simulink model "backstepping_HW"  (R2023a)
settings: Solver=FixedStepAuto  StartTime=0.0  StopTime=inf  FixedStep=0.001  RelTol=1e-3  EnableMultiTasking=on
values from neighbouring files (symbols this model uses):
  R_p_x = sqrt(2)/2*[-1 1 ... (first row only)    [Init_control.m]
undefined symbols (not defined in the file or in its folder): dev, Main, pwm_output0
libraries: px4Sensorslib x2, simulink x2, px4lib x1
settings Model: SimulationMode=external  ExtModeTrigDuration=10  Creator=ArriGE66  LastModifiedBy=matte
settings SolverCC: PositivePriorityOrder=on
settings OptimizationCC: EnhancedBackFolding=on  PassReuseOutputArgsAs=Individual arguments  ZeroExternalMemoryAtStartup=off  ZeroInternalMemoryAtStartup=off  MaxStackSize=64  OptimizeBlockOrder=speed  DifferentSizesBufferReuse=on  EfficientTunableParamExpr=on
settings DebuggingCC: ParameterTunabilityLossMsg=error
settings HardwareCC: ProdBitPerPointer=32  ProdBitPerSizeT=32  ProdBitPerPtrDiffT=32  ProdLargestAtomicInteger=Long  ProdLargestAtomicFloat=Double  ProdWordSize=32  ProdLongLongMode=on  ProdHWDeviceType=ARM Compatible->ARM Cortex
settings SFSimCC: MATLABDynamicMemAlloc=off  SimTargetLang=C++
settings RTWCC: Description=Embedded Coder  SystemTargetFile=ert.tlc  HardwareBoard=PX4 Cube Orange  TemplateMakefile=ert_default_tmf  Toolchain=GNU Tools for PX4 Autopilots  TargetLang=C++
settings CodeAppCC: ForceParamTrailComments=on  IgnoreCustomStorageClasses=off  OperatorAnnotations=on  SimulinkDataObjDesc=on  SFDataObjDesc=on  InsertBlockDesc=on
settings ERTTargetCC: ExtMode=on  ExtModeTransport=3  ExtModeStaticAlloc=on  ExtModeStaticAllocSize=1024  ExtModeMexFile=ext_xcp  ExtModeMexArgs=1 COM10 3000000  ExtModeIntrfLevel=Level2 - Open

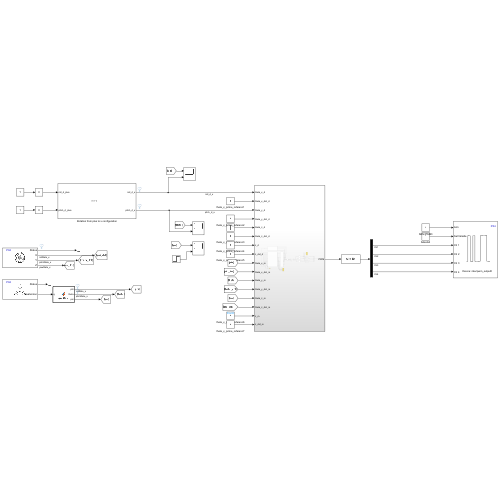
[thumbnail: Simulink's stored preview of the top-level diagram]
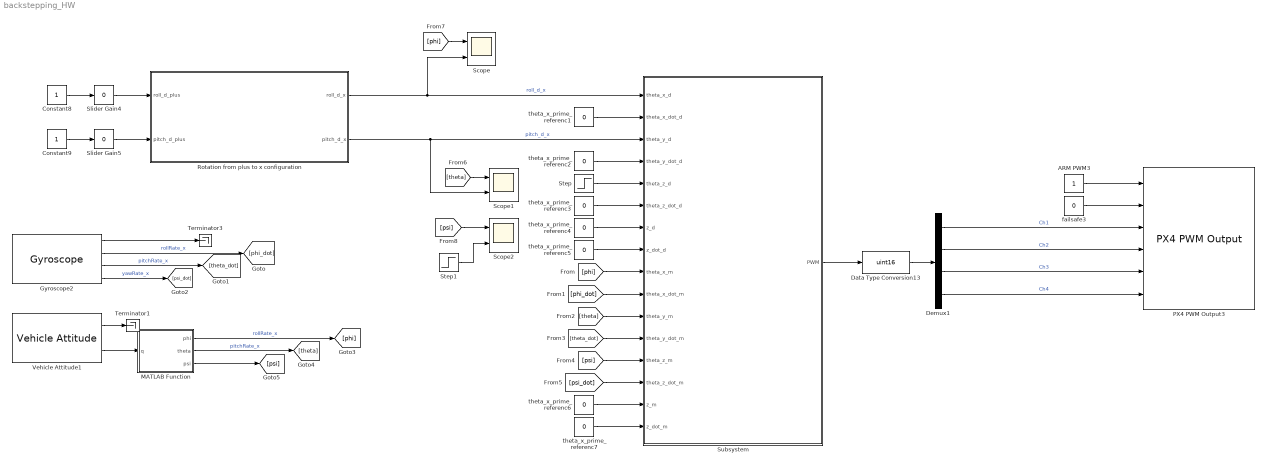
== system backstepping_HW ==
  ARM PWM3 : Constant  OutDataTypeStr=boolean  SampleTime=0.002
  Constant8 : Constant  SampleTime=-1
  Constant9 : Constant  SampleTime=-1
  Data Type Conversion13 : DataTypeConversion  OutDataTypeStr=uint16  SaturateOnIntegerOverflow=off  RndMeth=Floor
  Demux1 : Demux
  Gyroscope2 : px4Sensorslib/Gyroscope  uorbTimeStamp=off  BlockingMode=off  BlockTimeout=1e-3  sampleTime=0.002
  MATLAB Function : MATLAB Function  TreatAsAtomicUnit=on
  PX4 PWM Output3 : px4lib/PX4 PWM Output  pwmDevice=Main (/dev/pwm_output0)  pwmChannel1_=on  pwmChannel2_=on  pwmChannel3_=on  pwmChannel4_=on  pwmChannel5_=off  pwmChannel6_=off  pwmChannel7_=off  pwmChannel8_=off  forceTerminateFailsafe=off  outputErrorStatus=off
  Rotation from plus to x configuration : Subsystem
      mask Display: image('rotation_matrix.jpg');
  Scope : Scope  NumInputPorts=2
  Scope1 : Scope  NumInputPorts=2
  Scope2 : Scope  NumInputPorts=2
  Slider Gain4 : simulink/Math Operations/Slider Gain  gain=0  low=0  high=0.5
  Slider Gain5 : simulink/Math Operations/Slider Gain  gain=0  low=0  high=0.5
  Step : Step  After=0.6085  SampleTime=0.002
  Step1 : Step  After=0.6085  SampleTime=0.002
  Subsystem : Subsystem
  Terminator1 : Terminator
  Terminator3 : Terminator
  Vehicle Attitude1 : px4Sensorslib/Vehicle Attitude  rollRate=off  pitchRate=off  yawRate=off  quaternion=on  uorbTimeStamp=off  BlockingMode=off  BlockTimeout=0.001  sampleTime=0.002
  failsafe3 : Constant  Value=0  OutDataTypeStr=boolean  SampleTime=0.002
  theta_x_prime_referenc{1..7} (7 alike) : Constant  Value=0  SampleTime=0.002
  wires:
  Subsystem/1(PWM) -> Data Type Conversion13/1
  Data Type Conversion13/1 -> Demux1/1
  Demux1/1 -> PX4 PWM Output3/3  "Ch1"
  Demux1/2 -> PX4 PWM Output3/4  "Ch2"
  ARM PWM3/1 -> PX4 PWM Output3/1
  failsafe3/1 -> PX4 PWM Output3/2
  Vehicle Attitude1/2 -> MATLAB Function/1(q)
  Step/1 -> Subsystem/5(theta_z_d)
  Demux1/3 -> PX4 PWM Output3/5  "Ch3"
  Demux1/4 -> PX4 PWM Output3/6  "Ch4"
  Vehicle Attitude1/1 -> Terminator1/1
  Gyroscope2/1 -> Terminator3/1
  Rotation from plus to x configuration/2(pitch_d_x) -> Subsystem/3(theta_y_d), Scope1/2  "pitch_d_x"
  Rotation from plus to x configuration/1(roll_d_x) -> Scope/2, Subsystem/1(theta_x_d)  "roll_d_x"
  theta_x_prime_referenc1/1 -> Subsystem/2(theta_x_dot_d)
  theta_x_prime_referenc2/1 -> Subsystem/4(theta_y_dot_d)
  theta_x_prime_referenc3/1 -> Subsystem/6(theta_z_dot_d)
  theta_x_prime_referenc4/1 -> Subsystem/7(z_d)
  theta_x_prime_referenc5/1 -> Subsystem/8(z_dot_d)
  theta_x_prime_referenc6/1 -> Subsystem/15(z_m)
  theta_x_prime_referenc7/1 -> Subsystem/16(z_dot_m)
  Constant8/1 -> Slider Gain4/1
  Slider Gain4/1 -> Rotation from plus to x configuration/1(roll_d_plus)
  Constant9/1 -> Slider Gain5/1
  Slider Gain5/1 -> Rotation from plus to x configuration/2(pitch_d_plus)
  Gyroscope2/2 -> [phi_dot]  "rollRate_x"
  Gyroscope2/3 -> [theta_dot]  "pitchRate_x"
  Gyroscope2/4 -> [psi_dot]  "yawRate_x"
  MATLAB Function/1(phi) -> [phi]  "rollRate_x"
  MATLAB Function/2(theta) -> [theta]  "pitchRate_x"
  MATLAB Function/3(psi) -> [psi]
  [phi] -> Subsystem/9(theta_x_m)
  [phi_dot] -> Subsystem/10(theta_x_dot_m)
  [theta] -> Subsystem/11(theta_y_m)
  [theta_dot] -> Subsystem/12(theta_y_dot_m)
  [psi] -> Subsystem/13(theta_z_m)
  [psi_dot] -> Subsystem/14(theta_z_dot_m)
  [theta] -> Scope1/1
  [phi] -> Scope/1
  Step1/1 -> Scope2/2
  [psi] -> Scope2/1

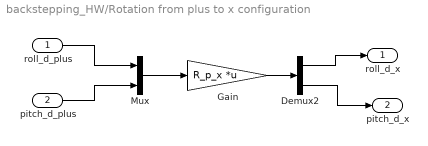
== system backstepping_HW/Rotation from plus to x configuration ==
  roll_d_plus : Inport
  pitch_d_plus : Inport  Port=2
  Demux2 : Demux  Outputs=2
  Gain : Gain  Gain=R_p_x  Multiplication=Matrix(K*u) (u vector)
  Mux : Mux  Inputs=2
  roll_d_x : Outport
  pitch_d_x : Outport  Port=2
  wires:
  roll_d_plus/1 -> Mux/1
  Mux/1 -> Gain/1
  Demux2/1 -> roll_d_x/1
  Gain/1 -> Demux2/1
  pitch_d_plus/1 -> Mux/2
  Demux2/2 -> pitch_d_x/1

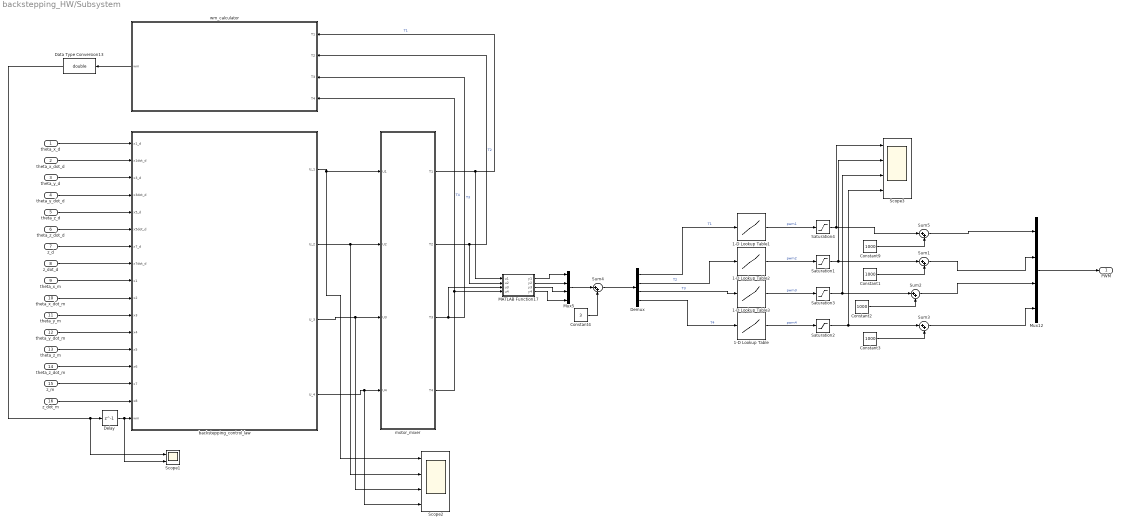
== system backstepping_HW/Subsystem ==
  theta_x_d : Inport
  theta_x_dot_d : Inport  Port=2
  theta_y_d : Inport  Port=3
  theta_y_dot_d : Inport  Port=4
  theta_z_d : Inport  Port=5
  theta_z_dot_d : Inport  Port=6
  z_d : Inport  Port=7
  z_dot_d : Inport  Port=8
  theta_x_m : Inport  Port=9
  theta_x_dot_m : Inport  Port=10
  theta_y_m : Inport  Port=11
  theta_y_dot_m : Inport  Port=12
  theta_z_m : Inport  Port=13
  theta_z_dot_m : Inport  Port=14
  z_m : Inport  Port=15
  z_dot_m : Inport  Port=16
  1-D Lookup Table : Lookup_n-D  NumberOfTableDimensions=1  BreakpointsForDimension1=[0;0.06477642396;0.16;0.63;2.44;4.43;6.92;8.77;10.52;11.63;12.03;12.09;12.091;12.092;12.093;12.094;12.095;12.096;12.097;12.098;12.099]  Table=[0;50;100;150;200;250;300;350;400;450;500;550;600;650;700;750;800;850;900;950;1000]  InternalRulePriority=Speed  RndMeth=Simplest
  1-D Lookup Table1 : Lookup_n-D  NumberOfTableDimensions=1  BreakpointsForDimension1=[0;0.02;0.06;0.29;0.73;1.07;1.88;2.91;4;5.06;6.71;7.86;9.41;10.86;11.45;11.82;12.07;12.31;12.52;12.74;12.75]  Table=[0;50;100;150;200;250;300;350;400;450;500;550;600;650;700;750;800;850;900;950;1000]  InternalRulePriority=Speed  RndMeth=Simplest
  1-D Lookup Table2 : Lookup_n-D  NumberOfTableDimensions=1  BreakpointsForDimension1=[0;0.05;0.39;1.67;3.19;5.57;8.07;10.01;10.71;11.06;11.42;11.53;11.55;11.551;11.552;11.553;11.554;11.555;11.556;11.557;11.558]  Table=[0;50;100;150;200;250;300;350;400;450;500;550;600;650;700;750;800;850;900;950;1000]  InternalRulePriority=Speed  RndMeth=Simplest
  1-D Lookup Table3 : Lookup_n-D  NumberOfTableDimensions=1  BreakpointsForDimension1=[0;0.06;0.23;0.89;2.47;3.9;5.86;7.81;9.42;10.12;10.6;11.01;11.34;11.39;11.391;11.392;11.393;11.394;11.395;11.396;11.397]  Table=[0;50;100;150;200;250;300;350;400;450;500;550;600;650;700;750;800;850;900;950;1000]  InternalRulePriority=Speed  RndMeth=Simplest
  Constant{1..3,9} (4 alike) : Constant  Value=1000  SampleTime=-1
  Constant4 : Constant  Value=3
  Data Type Conversion13 : DataTypeConversion  OutDataTypeStr=double  SaturateOnIntegerOverflow=off  RndMeth=Floor
  Delay : Delay  DelayLength=1
  Demux : Demux
  MATLAB Function17 : MATLAB Function  TreatAsAtomicUnit=on
  Mux12 : Mux
  Mux5 : Mux
  Saturation{1..4} (4 alike) : Saturate  UpperLimit=1000  LowerLimit=0
  Scope1 : Scope  NumInputPorts=2
  Scope2 : Scope  NumInputPorts=4
  Scope3 : Scope  NumInputPorts=4
  Sum{1..5} (5 alike) : Sum  Inputs=|++
  backstepping_control_law : MATLAB Function  TreatAsAtomicUnit=on
  motor_mixer : MATLAB Function  SystemSampleTime=0.004
  wm_calculator : MATLAB Function  TreatAsAtomicUnit=on
  PWM : Outport  VectorParamsAs1DForOutWhenUnconnected=off
  wires:
  theta_x_d/1 -> backstepping_control_law/1(x1_d)
  theta_x_dot_d/1 -> backstepping_control_law/2(x1dot_d)
  theta_y_d/1 -> backstepping_control_law/3(x3_d)
  theta_y_dot_d/1 -> backstepping_control_law/4(x3dot_d)
  theta_z_d/1 -> backstepping_control_law/5(x5_d)
  theta_z_dot_d/1 -> backstepping_control_law/6(x5dot_d)
  theta_x_m/1 -> backstepping_control_law/9(x1)
  theta_x_dot_m/1 -> backstepping_control_law/10(x2)
  theta_y_m/1 -> backstepping_control_law/11(x3)
  theta_y_dot_m/1 -> backstepping_control_law/12(x4)
  theta_z_m/1 -> backstepping_control_law/13(x5)
  theta_z_dot_m/1 -> backstepping_control_law/14(x6)
  Mux12/1 -> PWM/1
  backstepping_control_law/3(U_3) -> Scope2/3, motor_mixer/3(U3)
  backstepping_control_law/4(U_4) -> Scope2/4, motor_mixer/4(U4)
  wm_calculator/1(wm) -> Data Type Conversion13/1
  z_d/1 -> backstepping_control_law/7(x7_d)
  z_dot_d/1 -> backstepping_control_law/8(x7dot_d)
  z_m/1 -> backstepping_control_law/15(x7)
  z_dot_m/1 -> backstepping_control_law/16(x8)
  motor_mixer/4(T4) -> MATLAB Function17/4(u4), wm_calculator/4(T4)  "T4"
  1-D Lookup Table3/1 -> Saturation3/1  "pwm3"
  motor_mixer/1(T1) -> MATLAB Function17/1(u1), wm_calculator/1(T1)  "T1"
  motor_mixer/3(T3) -> MATLAB Function17/3(u3), wm_calculator/3(T3)  "T3"
  1-D Lookup Table2/1 -> Saturation1/1  "pwm2"
  1-D Lookup Table1/1 -> Saturation4/1  "pwm1"
  motor_mixer/2(T2) -> MATLAB Function17/2(u2), wm_calculator/2(T2)  "T2"
  Sum5/1 -> Mux12/1
  Saturation4/1 -> Scope3/1, Sum5/1
  Constant9/1 -> Sum5/2
  1-D Lookup Table/1 -> Saturation2/1  "pwm4"
  Saturation1/1 -> Scope3/2, Sum1/1
  Sum1/1 -> Mux12/2
  Constant1/1 -> Sum1/2
  Saturation3/1 -> Scope3/3, Sum2/1
  Sum2/1 -> Mux12/3
  Constant2/1 -> Sum2/2
  Saturation2/1 -> Scope3/4, Sum3/1
  Sum3/1 -> Mux12/4
  Constant3/1 -> Sum3/2
  Delay/1 -> Scope1/2, backstepping_control_law/17(wm)
  backstepping_control_law/1(U_1) -> Scope2/1, motor_mixer/1(U1)
  backstepping_control_law/2(U_2) -> Scope2/2, motor_mixer/2(U2)
  Data Type Conversion13/1 -> Delay/1, Scope1/1
  Constant4/1 -> Sum4/2
  Demux/3 -> 1-D Lookup Table3/1  "T3"
  Sum4/1 -> Demux/1
  Mux5/1 -> Sum4/1
  MATLAB Function17/3(y3) -> Mux5/3
  MATLAB Function17/1(y1) -> Mux5/1
  MATLAB Function17/4(y4) -> Mux5/4
  Demux/4 -> 1-D Lookup Table/1  "T4"
  MATLAB Function17/2(y2) -> Mux5/2
  Demux/2 -> 1-D Lookup Table2/1  "T2"
  Demux/1 -> 1-D Lookup Table1/1  "T1"

== matlab function backstepping_HW/Subsystem/wm_calculator ==
  data: T1 input; wm output; T2 input; T3 input; T4 input; quadParams parameter
function wm = wm_calculator(T1,T2,T3,T4,quadParams)

wm1=sqrt(abs(T1/quadParams.kd));
wm2=sqrt(abs(T2/quadParams.kd));
wm3=sqrt(abs(T3/quadParams.kd));
wm4=sqrt(abs(T4/quadParams.kd));


% da cambiare in base al nostro modello
wm=wm1+wm2-wm3-wm4;

== matlab function backstepping_HW/Subsystem/backstepping_control_law ==
  data: x1_d input; U_1 output; x1dot_d input; x3_d input; x3dot_d input; x5_d input; x5dot_d input; x7_d input; x7dot_d input; x1 input; x2 input; x3 input; x4 input; x5 input; x6 input; x7 input; x8 input; U_2 output; U_3 output; wm input; quadParams parameter; U_4 output
function [U_1,U_2,U_3,U_4] = backstepping_control_law(x1_d,x1dot_d,x3_d,x3dot_d,x5_d,x5dot_d,x7_d,x7dot_d,x1,x2,x3,x4,x5,x6,x7,x8,wm,quadParams)

alpha_angle=50; %va fatto il tuning di questo, devono essere costanti > 0
alpha_angleRate=1\10;

alpha1=alpha_angle;
alpha2=alpha_angleRate;
alpha3=alpha_angle;
alpha4=alpha_angleRate;
alpha5=alpha_angle;
alpha6=alpha_angleRate;
alpha7=alpha_angle;
alpha8=alpha_angleRate;




a1=(quadParams.Jy-quadParams.Jz)/quadParams.Jx;
a2=-quadParams.Jr/quadParams.Jx;
a3=(quadParams.Jz-quadParams.Jx)/quadParams.Jy;
a4=quadParams.Jr/quadParams.Jy;
a5=(quadParams.Jx-quadParams.Jy)/quadParams.Jz;
b1=quadParams.L/quadParams.Jx;
b2=quadParams.L/quadParams.Jy;
b3=quadParams.L/quadParams.Jz;



% LEGEND
% x1=theta_x;
% x2=theta_x_dot;
% x3=theta_y;
% x4=theta_y_dot;
% x5=theta_z;
% x6=theta_z_dot;
% x7=z;
% x8=z_dot;






z1=x1_d-x1;
z2=x2-x1dot_d-alpha1*z1;
z3=x3_d-x3;
z4=x4-x3dot_d-alpha3*z3;
z5=x5_d-x5;
z6=x6-x5dot_d-alpha5*z5;
z7=x7_d-x7;
z8=x8-x7dot_d-alpha7*z7;


U_2=(z1-a1*x4*x6-a2*x4*wm-alpha1*(z2+alpha1*z1)-alpha2*z2)/b1;
U_3=(z3-a3*x2*x6-a4*x2*wm-alpha3*(z4+alpha3*z3)-alpha4*z4)/b2;
U_4=(z5-a5*x2*x4-alpha5*(z6+alpha5*z5)-alpha6*z6)/b3;
U_1=quadParams.m*(z7+quadParams.g-alpha7*(z8+alpha7*z7)-alpha8*z8)/(cos(x1)*cos(x3));

== matlab function backstepping_HW/MATLAB Function ==
  data: q input; phi output; theta output; psi output
function [phi,theta,psi] = quat2eul(q)
% Conversion from Quaternion to Euler angles based on the PX4 Firmware
% v1.6.5 release.
% 
% Quaternion -> DCM -> Euler Angles
% INPUT:
%   q: Quaternion vector of the format: (a + bi + cj + dk)
% OUTPUT:
%   [phi,theta,psi]: Euler angles in radians.
% 
 
    a = q(1);
    b = q(2);
    c = q(3);
    d = q(4);

    aSq = a*a;
    bSq = b*b;
    cSq = c*c;
    dSq = d*d;

    d_pi2 = pi/2;

    % quaternion_to_dcm
    dcm00 = aSq + bSq - cSq - dSq;
    % dcm01 = 2*(b*c - a*d);
    dcm02 = 2*(a*c + b*d);
    dcm10 = 2*(b*c + a*d);
    % dcm11 = aSq - bSq + cSq - dSq;
    dcm12 = 2*(c*d - a*b);
    dcm20 = 2*(b*d - a*c);
    dcm21 = 2*(a*b + c*d);
    dcm22 = aSq - bSq - cSq + dSq;

    % dcm_to_euler
    theta = asin(-dcm20);
    if abs(theta - d_pi2) < 1.0e-3
        phi = single(0.0);
        psi = atan2(dcm12, dcm02);
    elseif abs(theta + d_pi2) < 1.0e-3
        phi = single(0.0);
        psi = atan2(-dcm12, -dcm02);
    else
        phi = atan2(dcm21, dcm22);
        psi = atan2(dcm10, dcm00);
    end

end

== matlab function backstepping_HW/Subsystem/motor_mixer ==
  data: U1 input; T1 output; U2 input; U3 input; U4 input; T2 output; T3 output; T4 output; quadParams parameter
function [T1,T2,T3,T4] = motor_mixer(U1,U2,U3,U4,quadParams)
%Function description:
%  Control allocation. The quadrotor type is X-configuration,
%  and the airframe is as follows:
%3↓   1↑
 %  \ /
 %  / \
 %2↑   4↓


% |U1|    |       1             1           1            1       |  |T1|
% |U2|  = | -L*sqrt(2)/2  L*sqrt(2)/2  L*sqrt(2)/2  -L*sqrt(2)/2 |  |T2|
% |U3|    | L*sqrt(2)/2  -L*sqrt(2)/2  L*sqrt(2)/2  -L*sqrt(2)/2 |  |T3| 
% |U4|    | kd/kt            kd/kt       -kd/kt       -kd/kt     |  |T4|



% we need to invert this in order to obtain 
% |T1|                              |U1|
% |T2| =  quadParams.MotorMixer *   |U2|
% |T3|                              |U3|
% |T4|                              |U4|

U=[U1;U2;U3;U4];
T=quadParams.MotorMixer*U;
T1=T(1);
T2=T(2);
T3=T(3);
T4=T(4);

== matlab function backstepping_HW/Subsystem/MATLAB Function17 ==
  data: u1 input; y1 output; u2 input; u3 input; u4 input; y2 output; y3 output; y4 output
function [y1,y2,y3,y4] = fcn(u1,u2,u3,u4)

if u1 < 0
    u2 = u2 + abs(u1);
    u1 = u1+abs(u1);
end
if u2 < 0
    u2 = u2 + abs(u2);
    u1 = u1 + abs(u2);
end
if u3 < 0
    u3 = u3 + abs(u3);
    u4 = u4 + abs(u3);
end    
if u4 < 0
    u4 = u4 + abs(u4);
    u3 = u3 + abs(u4);
end
 y1 = u1;
 y2 = u2;
 y3 = u3;
 y4 = u4;
